simulink model "testUDP"  (R2018b)
settings: Solver=FixedStepAuto  StartTime=0.0  StopTime=40  FixedStep=0.0125  RelTol=1e-3  EnableMultiTasking=on
values from neighbouring files (symbols this model uses):
  dynamicsRate = 0.0125    [loadBusData.m]
settings Model: Creator=barthal  LastModifiedBy=barthal
settings SolverCC: PositivePriorityOrder=on
settings DataIOCC: Decimation=5  SaveFormat=StructureWithTime
settings OptimizationCC: EnhancedBackFolding=on  PassReuseOutputArgsAs=Individual arguments  MaxStackSize=64  OptimizeBlockOrder=speed  DifferentSizesBufferReuse=on  OptimizationCustomize=off
settings DebuggingCC: ParameterTunabilityLossMsg=error
settings HardwareCC: ProdBitPerPointer=32  ProdBitPerSizeT=32  ProdBitPerPtrDiffT=32  ProdLargestAtomicInteger=Long  ProdLargestAtomicFloat=Double  ProdWordSize=32  ProdHWDeviceType=ARM Compatible->ARM Cortex
settings ModelReferenceCC: ModelReferenceNumInstancesAllowed=Single
settings RTWCC: SystemTargetFile=ert.tlc  HardwareBoard=Raspberry Pi  TLCOptions="-aInlineSetEventsForThisBaseRateFcn=TLC_FALSE -aSuppressMultiTaskScheduler=TLC_FALSE  -aRateBasedStepFcn=0"  GenCodeOnly=on  TemplateMakefile=ert_default_tmf  GenerateReport=on  Toolchain=GNU GCC Raspberry Pi  BuildConfiguration=Faster Runs  IncludeHyperlinkInReport=on  LaunchReport=on  TargetLang=C++  GenerateTraceInfo=on  GenerateTraceReport=on  GenerateTraceReportSl=on  GenerateTraceReportSf=on  GenerateTraceReportEml=on
settings CodeAppCC: ForceParamTrailComments=on  IgnoreCustomStorageClasses=off  OperatorAnnotations=on  SimulinkDataObjDesc=on  SFDataObjDesc=on  InsertBlockDesc=on
settings ERTTargetCC: TargetLangStandard=C++03 (ISO)  MatFileLogging=on  MultiInstanceERTCode=on  CodeInterfacePackaging=C++ class  SupportVariableSizeSignals=on  MultiInstanceErrorCode=Warning  RootIOFormat=Structure reference

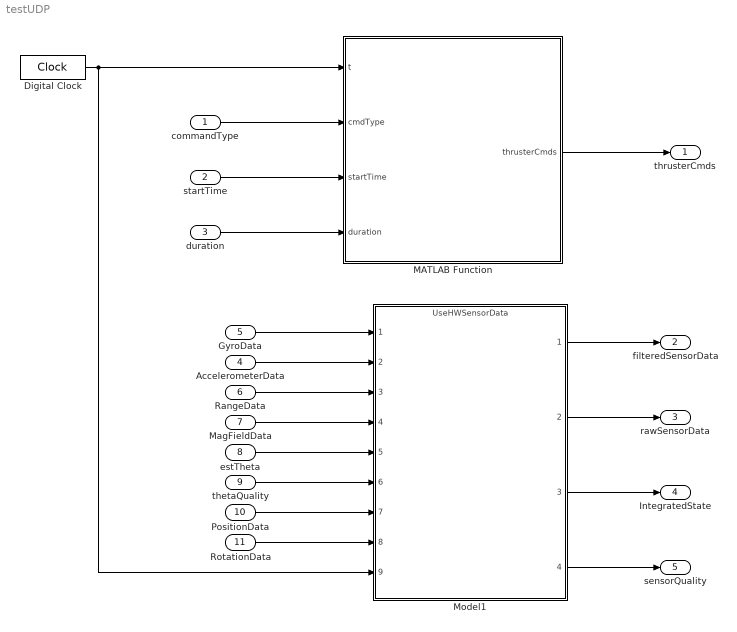
== system testUDP ==
  commandType : Inport  OutDataTypeStr=int32
  startTime : Inport  Port=2
  duration : Inport  Port=3
  AccelerometerData : Inport  Port=4  OutDataTypeStr=double  PortDimensions=3
  GyroData : Inport  Port=5  OutDataTypeStr=double  PortDimensions=3
  RangeData : Inport  Port=6  OutDataTypeStr=int32
  MagFieldData : Inport  Port=7
  estTheta : Inport  Port=8
  thetaQuality : Inport  Port=9
  PositionData : Inport  Port=10
  RotationData : Inport  Port=11
  Digital Clock : DigitalClock  SampleTime=dynamicsRate
  MATLAB Function : MATLAB Function  TreatAsAtomicUnit=on
  Model1 : ModelReference  ModelNameDialog=UseHWSensorData  SimulationMode=Normal  VariantControl=VSS_HWSENSOR  ModelReferenceVersion=1.145
  thrusterCmds : Outport
  filteredSensorData : Outport  Port=2  OutDataTypeStr=double
  rawSensorData : Outport  Port=3  OutDataTypeStr=double
  IntegratedState : Outport  Port=4  OutDataTypeStr=double
  sensorQuality : Outport  Port=5
  wires:
  MATLAB Function/1(thrusterCmds) -> thrusterCmds/1
  Digital Clock/1 -> Model1/9, MATLAB Function/1(t)
  commandType/1 -> MATLAB Function/2(cmdType)
  startTime/1 -> MATLAB Function/3(startTime)
  duration/1 -> MATLAB Function/4(duration)
  AccelerometerData/1 -> Model1/2
  GyroData/1 -> Model1/1
  RangeData/1 -> Model1/3
  MagFieldData/1 -> Model1/4
  estTheta/1 -> Model1/5
  thetaQuality/1 -> Model1/6
  PositionData/1 -> Model1/7
  RotationData/1 -> Model1/8
  Model1/1 -> filteredSensorData/1
  Model1/2 -> rawSensorData/1
  Model1/3 -> IntegratedState/1
  Model1/4 -> sensorQuality/1

== matlab function testUDP/MATLAB Function ==
  data: t input; thrusterCmds output; cmdType input; startTime input; duration input
function thrusterCmds = fcn(t,cmdType,startTime,duration)
%   Thruster Layout
%     3       2   
%    4         1
%
%
%    5         8       
%     6       7          ^
%                        | 
%  + X -->             + Y 

% cmdType firing axis
%    1 = +X Tran
%    2 = -X Tran
%    3 = +Y Tran
%    4 = -Y Tran
%    5 = +Z Rot 
%    6 = -Z Rot

% Default to zero each pass
thrusterCmds = zeros(1,8);
cmdNow = 0;

if t >= startTime
    if t < startTime+duration
        cmdNow = 1;
    end
end
   
if cmdNow == 1
    if cmdType == 1
        thrusterCmds(4) = 1;
        thrusterCmds(5) = 1;
    elseif cmdType == 2
        thrusterCmds(1) = 1;
        thrusterCmds(8) = 1;
    elseif cmdType == 3
        thrusterCmds(6) = 1;
        thrusterCmds(7) = 1;
    elseif cmdType == 4
        thrusterCmds(2) = 1;
        thrusterCmds(3) = 1;
    elseif cmdType == 5
        thrusterCmds(1) = 1;
        thrusterCmds(5) = 1;
    elseif cmdType == 6
        thrusterCmds(4) = 1;
        thrusterCmds(8) = 1;
    end
end
%     if mod(t,0.05) == 0
%         fprintf('Time is: %8.3f\n',t);
%     end
